simulink model "decoder"  (R2013b)
settings: Solver=FixedStepDiscrete  SolverMode=SingleTasking  StartTime=0  StopTime=8000  RelTol=1e-3
model workspace (MAT data in the model file):
  logicAddr = 2
settings Model: Creator=qiji  LastModifiedBy=qiji
settings DataIOCC: SaveOutput=off  SaveTime=off
settings OptimizationCC: BlockReduction=off  ConditionallyExecuteInputs=off  InlineParams=on
settings DebuggingCC: UnderspecifiedInitializationDetection=Simplified  MultiTaskDSMMsg=warning  MultiTaskCondExecSysMsg=none  SingleTaskRateTransMsg=error  SFUnusedDataAndEventsDiag=none
settings RTWCC: IncludeERTFirstTime=on
settings GRTTargetCC: CodeReplacementLibrary=None  CPPClassGenCompliant=on
settings ConfigurationSet: Description=SimMechanics 2G

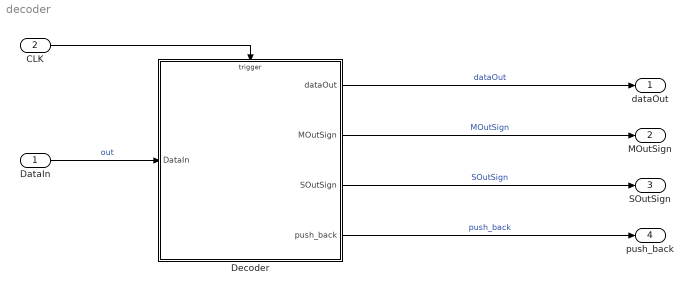
== system decoder ==
  DataIn : Inport  OutDataTypeStr=uint32  PortDimensions=1  SampleTime=[1,0]
  CLK : Inport  Port=2  OutDataTypeStr=boolean  PortDimensions=1  SampleTime=[1,0]
  Decoder : Stateflow chart  TreatAsAtomicUnit=on
  dataOut : Outport  OutDataTypeStr=uint32  PortDimensions=1  SampleTime=[1,0]
  MOutSign : Outport  Port=2  OutDataTypeStr=boolean  PortDimensions=1  SampleTime=[1,0]
  SOutSign : Outport  Port=3  OutDataTypeStr=boolean  PortDimensions=1  SampleTime=[1,0]
  push_back : Outport  Port=4  OutDataTypeStr=boolean  PortDimensions=1  SampleTime=[1,0]
  wires:
  CLK/1 -> Decoder/Trigger
  DataIn/1 -> Decoder/1(DataIn)  "out"
  Decoder/1(dataOut) -> dataOut/1  "dataOut"
  Decoder/4(push_back) -> push_back/1  "push_back"
  Decoder/2(MOutSign) -> MOutSign/1  "MOutSign"
  Decoder/3(SOutSign) -> SOutSign/1  "SOutSign"

== stateflow chart decoder/Decoder ==
  settings: executeAtInitialization=1  initializeOutput=1
  state judge_data [parallel]
    settings: executionOrder=1
    state MF
      en:
      MOutSign= true;
    state wait4Data
      en:
      [buffer, index] = initBuffer();
    state judgeData
      en:
      receive_complete = false;
    state end
    state SF
      en:
      SOutSign=true;
    judgeData -> MF [order 1] : [judge(buffer)==1]
    MF -> end
    wait4Data -> judgeData : [receive_complete == true]
    (default) -> wait4Data
    judgeData -> wait4Data [order 3] : [judge(buffer)==0]
    judgeData -> SF [order 2] : [judge(buffer)==2]
    end -> wait4Data
    SF -> end
  note: 0010//1100/0111/0001
      | 0101//0000/0000/0000
      | 0001//1010/1000/1110
      | 0000/0000/0011//0011
  state receiver [parallel]
    settings: executionOrder=2
    state decodeSF
      decodeSF -> decodeSF [order 1] : CLK
          | {
          | ans = bitoperate.shiftbit(ans, 1) + DataIn;
          | count++;
          | }
    note: 首先接受所有的数据，当接受完毕以后，再通知另外一个子系统判断
        | 从帧和主帧，并对dataout赋值。
    state judge
      en:
      ans = 0;
    state start
    decodeSF -> judge [order 1] : [count==32]
        | {
        | buffer[index] = ManchesterDecoding(ans);
        | count=0;
        | dataOut = buffer[index];
        | push_back = 1;
        | }
    start -> decodeSF : [DataIn == 1]
        | {
        | count = 2;
        | ans=1;
        | }
    judge -> decodeSF [order 1] : [!judgeEnd(buffer[index])]
        | {index++;}
    judge -> start [order 2] : {
        | receive_complete = true;
        | dataOut = 0;
        | }
    (default) -> start
  state bitoperate [group]
  data: r function_output double; dataBuffer function_input uint16 size=16; r function_output boolean; data function_input uint16; num function_input uint32; r function_output uint32; data function_input uint32; num function_input uint32; r function_output uint32; r function_output uint16 size=16; i function_output uint8; r function_output uint32; data function_input uint32; DataIn input uint32; dataOut output uint32; count local uint32; MOutSign output boolean; SOutSign output boolean; ans local uint32; buffer local uint16 size=16; index local uint8; push_back output boolean; receive_complete local boolean =false
  events: CLK input RISING_EDGE_EVENT
  function r = judge(dataBuffer):
    | function r = judge(dataBuffer)
    | low12 = bitshift(dataBuffer(1), 4);
    | high4 = bitshift(dataBuffer(2), -12);
    | start = low12 + high4;
    | r = 0;
    | if start == 50965
    |     r = 1;
    | elseif start == 43235
    |     r = 2;
    | end
  function r = judgeEnd(data):
    | function r = judgeEnd(data)
    | bit1 = bitget(data, 1);
    | bit2 = bitget(data, 2);
    | bit3 = bitget(data, 3);
    | bit4 = bitget(data, 4);
    | if bit1==1 && bit2==1 && bit3==0 && bit4==0
    |     r = true;
    | else
    |     r = false;
    | end
  function r = getbit(num):
    | function r = getbit(num)
    | r = bitget(num, 32);
  function r = shiftbit(data, num):
    | function r = shiftbit(data, num)
    | r = bitshift(data, num);
    | %for i=1:cnt
    | %   r = bitset(r, i, 0);
    | %end
  function [r, i] = initBuffer:
    | function [r, i] = initBuffer
    | r = [(uint16(0));(uint16(0));(uint16(0));(uint16(0));...
    |     (uint16(0));(uint16(0));(uint16(0));(uint16(0));...
    |     (uint16(0));(uint16(0));(uint16(0));(uint16(0));...
    |     (uint16(0));(uint16(0));(uint16(0));(uint16(0))];
    | i=uint8(0);
  function r = ManchesterDecoding(data):
    | function r = ManchesterDecoding(data)
    | r = uint32(0);
    | for i = (1:2:32)
    |     x0 = bitget(data, i);
    |     x1 = bitget(data, i+1);
    |     if x0==0 && x1==1
    |         r = bitset(r, (i+1)/2, 1);
    |     else
    |         r = bitset(r, (i+1)/2, 0);
    |     end
    | end
